simulink model "cart"  (Simulink 8.4)
settings: Solver=ode23  StartTime=0.0  StopTime=3  RelTol=1e-6
values from neighbouring files (symbols this model uses):
  a_max = 1    [assignment1.m]    (also in assignment3.m = p0 = -; assignment4.m = p0 = -)
  g3 = c2d(tf(1),h)    [assignment1.m]    (also in assignment3.m = c2d(tf(1,[tcAcc 1]),h,'tustin'); assignment4.m = c2d(tf(1,[tcAcc 1]),h,'tustin'); assignment5.m = c2d(tf(1,[tcAcc 1]),h,'tustin'); pend_init.m = c2d(tf(1,[tcAcc 1]),h,'tustin'))
  h = uIn(5*N+10)    [MPCsimulink.m]    (also in assignment1.m = 0.001; pend_init.m = 0.01)
  initPosError = 0    [assignment1.m]    (also in assignment3.m; assignment4.m; assignment5.m; pend_init.m)
  p0 = -1.5    [assignment1.m]    (also in assignment5.m = -0.8)
settings Model: Creator=pontusg  LastModifiedBy=frt090_B  ExtModeAutoUpdateStatusClock=off
settings OptimizationCC: InitFltsAndDblsToZero=on
settings DebuggingCC: SaveWithParameterizedLinksMsg=none
settings SFSimCC: SimParseCustomCode=off
settings GRTTargetCC: TargetFcnLib=ansi_tfl_tmw.mat

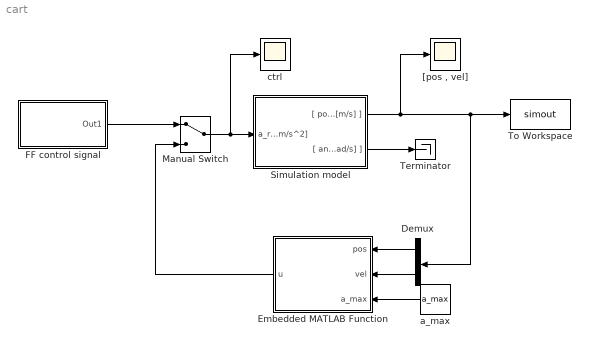
== system cart ==
  Demux : Demux  Outputs=2
  Embedded MATLAB Function : MATLAB Function  TreatAsAtomicUnit=on
  FF control signal : Subsystem
  Manual Switch : ManualSwitch
  Simulation model : Subsystem
  Terminator : Terminator
  To Workspace : ToWorkspace  VariableName=simout  SaveFormat=Structure With Time  SampleTime=-1
  "[pos , vel]" : Scope
  a_max : Constant  Value=a_max
  ctrl : Scope
  wires:
  Simulation model/1("[ pos [m] , vel [m/s] ]") -> To Workspace/1, Demux/1, "[pos , vel]"/1
  FF control signal/1(Out1) -> Manual Switch/1
  Manual Switch/1 -> ctrl/1, Simulation model/1(a_ref [m/s^2])
  Simulation model/2("[ ang [rad] , angVel [rad/s] ]") -> Terminator/1
  Embedded MATLAB Function/1(u) -> Manual Switch/2
  a_max/1 -> Embedded MATLAB Function/3(a_max)
  Demux/1 -> Embedded MATLAB Function/1(pos)
  Demux/2 -> Embedded MATLAB Function/2(vel)

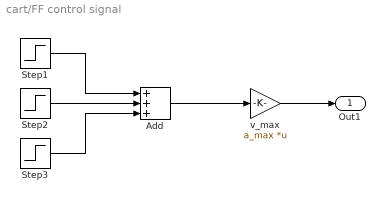
== system cart/FF control signal ==
  Add : Sum  Inputs=+++
  Step1 : Step  Time=0  SampleTime=0
  Step2 : Step  Time=t(1)  After=-2  SampleTime=0
  Step3 : Step  Time=t(2)  SampleTime=0
  v_max : Gain  Gain=a_max  Multiplication=Matrix(K*u) (u vector)
  Out1 : Outport
  wires:
  Add/1 -> v_max/1
  v_max/1 -> Out1/1
  Step1/1 -> Add/1
  Step2/1 -> Add/2
  Step3/1 -> Add/3

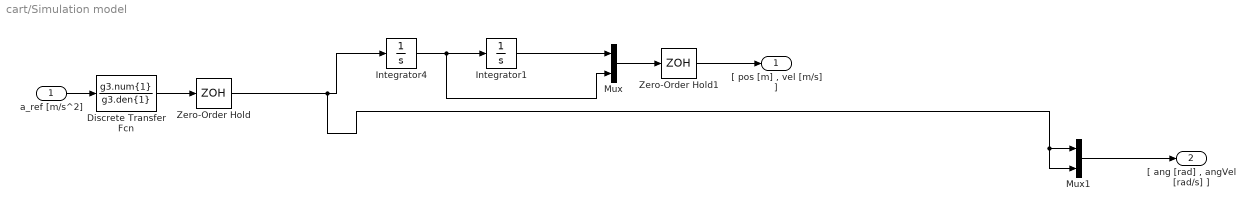
== system cart/Simulation model ==
  a_ref [m/s^2] : Inport
  Discrete Transfer Fcn : DiscreteTransferFcn  Numerator=g3.num{1}  Denominator=g3.den{1}  SampleTime=h
  Integrator1 : Integrator  InitialCondition=p0+initPosError
  Integrator4 : Integrator
  Mux : Mux  Inputs=2
  Mux1 : Mux  Inputs=2
  Zero-Order Hold : ZeroOrderHold  SampleTime=h
  Zero-Order Hold1 : ZeroOrderHold  SampleTime=h
  "[ pos [m] , vel [m/s] ]" : Outport
  "[ ang [rad] , angVel [rad/s] ]" : Outport  Port=2
  wires:
  Discrete Transfer Fcn/1 -> Zero-Order Hold/1
  a_ref [m/s^2]/1 -> Discrete Transfer Fcn/1
  Mux/1 -> Zero-Order Hold1/1
  Integrator1/1 -> Mux/1
  Integrator4/1 -> Mux/2, Integrator1/1
  Zero-Order Hold/1 -> Mux1/1, Mux1/2, Integrator4/1
  Zero-Order Hold1/1 -> "[ pos [m] , vel [m/s] ]"/1
  Mux1/1 -> "[ ang [rad] , angVel [rad/s] ]"/1

== matlab function Embedded MATLAB Function ==
  data: pos input double; u output double; vel input double; a_max input double
function u = fcn(pos,vel,a_max)
% pos is the position, vel is the velocity and a_max is a_max

% The if-clause is here to avoid chattering when close to the origin.
if ((pos/0.02)^2+(vel/0.1)^2>=0.3)
    u = 0;     % your controller goes here
else
    u = -3.12*pos-2.69*vel;  % to keep the cart at the origin, when close
end
